simulink subsystem "AutomaticTransmissionWithTorqueConverterSSC"  (R2025b)
settings: Solver=VariableStepAuto  StartTime=0.0  StopTime=10.0  RelTol=1e-3
undefined symbols (not defined in the file): Diff, Eng, PlntTransDampVect, PlntTransEffVect, PlntTransGearNumVect, PlntTransGearRatioVect, PlntTrqConvrtrImpDamp, PlntTrqConvrtrTurbDamp, Trans
libraries: fl_lib x11, sdl_lib x5, nesl_utility x4, nesl_utility_internal x3, autolibsharedcommon x1
settings Model: ModifiedByFormat=The MathWorks, Inc.  Creator=The MathWorks, Inc.  LastModifiedBy=The MathWorks, Inc.
settings OptimizationCC: ReuseModelBlockBuffer=off
settings DebuggingCC: SubsystemReferenceDiagnosticForUnitTest=warning
settings RTWCC: GPUComputeCapability=3.5

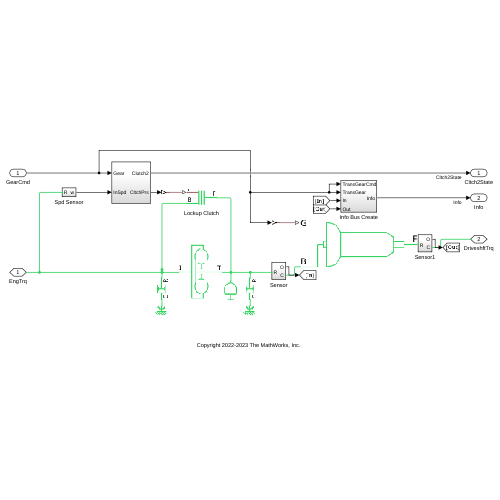
[thumbnail: Simulink's stored preview of the top-level diagram]
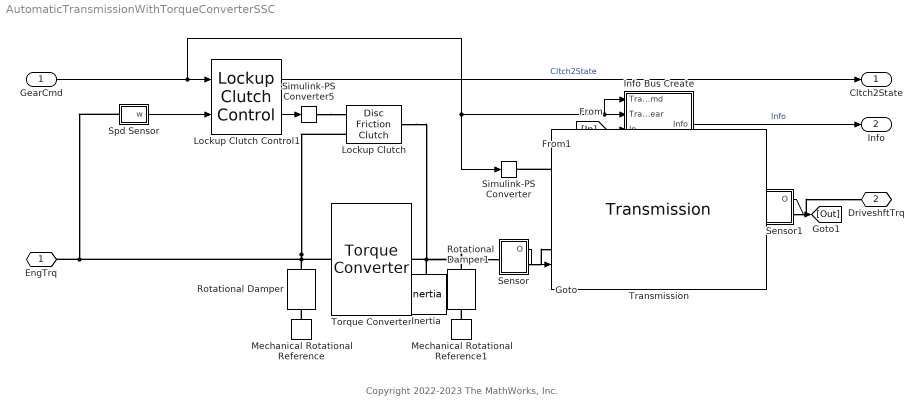
== system AutomaticTransmissionWithTorqueConverterSSC ==
  note: Copyright 2022-2023 The MathWorks, Inc.
  GearCmd : Inport
  Inertia : fl_lib/Mechanical/Rotational Elements/Inertia  inertia=PlntTrqConvrtrTurbInertia kg*m^2  num_ports=foundation.enum.numPorts2.one  w_specify=off  w_priority=High  w=0 rad/s  w_nominal_specify=off  w_nominal_value=1  w_nominal_unit=rad/s  t_specify=off  t_priority=None  t=0 N*m  t_nominal_specify=off  t_nominal_value=1  t_nominal_unit=N*m
  Info Bus Create : Subsystem
  Lockup Clutch : sdl_lib/Clutches/Disc Friction Clutch  geometry_model=sdl.enum.friction_geometry.radius  r_eff=PlntTrqConvrtrCltchRadius m  d_o=150 mm  d_i=100 mm  nS=PlntTrqConvrtrCltchNumFricSurf  piston_area=PlntTrqConvrtrCltchEngdPstnArea m^2  unidirectional=sdl.enum.directionality.bidirectional  friction_model=sdl.enum.friction_model_TLU_thermal.fixed  mu_w_vector=[0, 100, 1000] rad/s  temperature_TLU=[280, 300, 320] K  mu_static=PlntTrqConvrtrCltchStatFric  mu_static_vector=[.4, .38, .36]  mu_coulomb=PlntTrqConvrtrCltchKinFric  mu_coulomb_vector=[.3, .22, .19]  mu_coulomb_temp_vector=[.3, .28, .25]  mu_coulomb_matrix=[.34, .32, .3; .3, .28, .25; .25, .2, .15]  mu_interp_method=simscape.enum.interpolation.linear  mu_extrap_method=simscape.enum.extrapolation.linear  d_f=PlntTrqConvrtrCltchDerateFctr  w_tol=PlntTrqConvrtrCltchVelTol rad/s  pressure_min=PlntTrqConvrtrCltchEngdThreshPrs Pa  mu_visc=PlntTrqConvrtrCltchViscDragTrq N*m/(rad/s)  initial_state_locked=sdl.enum.initial_lock.unlocked  thermal_mass=25 kJ/K  T_init=300 K
      settings: InternalSimscapePortConfiguration="{\"Bottom\":[],\"Left\":[{\"id\":\"P\",\"label\":\"P\",\"type\":\"input\"},{\"id\":\"B\",\"label\":\"B\",\"type\":\"foundation.mechanical.rotational.rotational\"}],\"Right\":[{\"id\":\"F\",\"label\":\"F\",\"type\":\"foundation.mechanical.rotational.rotational\"}],\"Top\":[]}"
  Lockup Clutch Control1 : autolibsharedcommon/Lockup Clutch Control  SystemSampleTime=-1  VariantActivationTime=update diagram  EmptyChoice=off  PassThrough=off  PassThroughVariantControl=(default)  EmptyChoiceVariantControl=(default)  AllowFlexibleInterface=on  Latency=0  AutoFrameSizeCalculation=off
  Mechanical Rotational Reference : fl_lib/Mechanical/Rotational Elements/Mechanical Rotational Reference
  Mechanical Rotational Reference1 : fl_lib/Mechanical/Rotational Elements/Mechanical Rotational Reference
  Rotational Damper : sdl_lib/Couplings & Drives/Springs & Dampers/Rotational Damper  D=PlntTrqConvrtrImpDamp N*m*s/rad  thermal_port=simscape.enum.thermaleffects.omit  thermal_mass=50 kJ/K  temperature_specify=off  temperature_priority=High  temperature=300 K  temperature_nominal_specify=off  temperature_nominal_value=1  temperature_nominal_unit=K
  Rotational Damper1 : sdl_lib/Couplings & Drives/Springs & Dampers/Rotational Damper  D=PlntTrqConvrtrTurbDamp N*m*s/rad  thermal_port=simscape.enum.thermaleffects.omit  thermal_mass=50 kJ/K  temperature_specify=off  temperature_priority=High  temperature=300 K  temperature_nominal_specify=off  temperature_nominal_value=1  temperature_nominal_unit=K
  Sensor : Subsystem
  Sensor1 : Subsystem
  Simulink-PS Converter : nesl_utility_internal/Simulink-PS Converter  PhysicalDomain=network_engine_domain  SubClassName=ps_input  LeftPortType=input  RightPortType=output  PseudoPeriodic=off  Frequencies=[]  NoiseDistribution=none  NoiseParameters=[]  Unit=1  AffineConversion=off  FilteringAndDerivatives=provide  SimscapeFilterOrder=1  InputFilterTimeConstant=0.001  UdotUserProvided=0
  Simulink-PS Converter5 : nesl_utility_internal/Simulink-PS Converter  PhysicalDomain=network_engine_domain  SubClassName=ps_input  LeftPortType=input  RightPortType=output  PseudoPeriodic=off  Frequencies=[]  NoiseDistribution=none  NoiseParameters=[]  Unit=Pa  AffineConversion=off  FilteringAndDerivatives=provide  SimscapeFilterOrder=1  InputFilterTimeConstant=0.01  UdotUserProvided=0
  Spd Sensor : Subsystem
  Torque Converter : sdl_lib/Couplings & Drives/Torque Converter  coast_mode_modeling=sdl.enum.torqueConverterContinuousTwomode.continuous  SR_drive_tlu=PlntTrqConvrtrDrvModeSpdRatioVect  TR_drive_tlu=PlntTrqConvrtrDrvModeTrqRatioVect  CF_drive_tlu=PlntTrqConvrtrDrvModeCapFctrVect N*m/rpm^2  SR_coast_tlu=PlntTrqConvrtrCoastModeSpdRatioVect  CF_coast_tlu=PlntTrqConvrtrCoastModeCapFctrRatioVect N*m/rpm^2  iniMode=sdl.enum.torqueConverterInitialMode.drive  delta_w=PlntTrqConvrtrModeTransThresh rpm  n_vector=PlntTrqConvrtrSpdRatioVect  trq_vector=PlntTrqConvrtrTrqRatioVect  cf_vector_parameterization=sdl.enum.torqueConverterCFParameterization.SpeedToSqrtTorque  cf_vector_reference_speed=sdl.enum.torqueConverterCFReferenceSpeed.ImpellerSpeedAlways  cf_vector=PlntTrqConvrtrCapVect rad/(N^(1/2)*m^(1/2)*s)  cf_vector_sq=1e-3 * [6.616, 6.048, 5.787, 5.384, 4.681, 3.779, 2.671, 2.047, 1.111, .4] N*m*s^2/rad^2  interp_method=simscape.enum.interpolation.smooth  extrap_method=simscape.enum.extrapolation.nearest  model_lag=sdl.enum.torqueConverterLagOnOff.LagOff  tau=PlntTrqConvrtrTimeCnst s  initial_trq_ratio=PlntTrqConvrtrInitTrqRatio
      settings: InternalSimscapePortConfiguration="{\"Bottom\":[],\"Left\":[{\"id\":\"I\",\"label\":\"I\",\"type\":\"foundation.mechanical.rotational.rotational\"}],\"Right\":[{\"id\":\"T\",\"label\":\"T\",\"type\":\"foundation.mechanical.rotational.rotational\"}],\"Top\":[]}"
  Transmission : sdl_lib/Gears/Transmission  gear_ratios=PlntTransGearRatioVect(2:end)  reverse_ratio=PlntTransRvrseGearRatio  friction_model=sdl.enum.transmissionFriction.gear  efficiency=0.95  efficiency_tlu=PlntTransEffVect(2:end)  reverse_efficiency=PlntTransRvrseGearEff  pwr_thr=PlntTransPwrThresh W  kp=PlntTransStiff N*m/rad  kv=PlntTransDamp N*m*s/rad  initial_torque=PlntTransInitInTrq N*m  mu_visc=[PlntTransDampVect(1), PlntTransDampVect(1)] N*m*s/rad  t_friction=PlntTransCltchKinFricTrq N*m  t_locked=PlntTransCltchStatFricTrq N*m  shift_model=sdl.enum.transmissionShiftModel.instant  shift_time=PlntTransCltchShiftTime ms  w_tol=PlntTransCltchVelTol rad/s  initial_state_locked=sdl.enum.initial_lock.locked  thermal_port=simscape.enum.thermaleffects.omit  thermal_mass=100 kJ/K  initial_temperature=300 K
      settings: LogSimulationData=on  InternalSimscapePortConfiguration="{\"Bottom\":[],\"Left\":[{\"id\":\"G\",\"label\":\"G\",\"type\":\"input\"},{\"id\":\"B\",\"label\":\"B\",\"type\":\"foundation.mechanical.rotational.rotational\"}],\"Right\":[{\"id\":\"F\",\"label\":\"F\",\"type\":\"foundation.mechanical.rotational.rotational\"}],\"Top\":[]}"
  EngTrq : PMIOPort  Side=Left
  DriveshftTrq : PMIOPort  Port=2  Side=Right
  Cltch2State : Outport  VectorParamsAs1DForOutWhenUnconnected=off
  Info : Outport  Port=2  VectorParamsAs1DForOutWhenUnconnected=off
  wires:
  Info Bus Create/1(Info) -> Info/1  "Info"
  Lockup Clutch Control1/1 -> Cltch2State/1  "Cltch2State"
  GearCmd/1 -> Lockup Clutch Control1/1, Info Bus Create/2(TransGear), Info Bus Create/1(TransGearCmd), Simulink-PS Converter/1
  Lockup Clutch Control1/2 -> Simulink-PS Converter5/1
  Spd Sensor/1(w) -> Lockup Clutch Control1/2
  Sensor/1(O) -> [In]
  Sensor1/1(O) -> [Out]
  [In] -> Info Bus Create/3(In)
  [Out] -> Info Bus Create/4(Out)
  connections:
  Lockup Clutch/LConn2 -- EngTrq/RConn1 -- Spd Sensor/LConn1 -- Torque Converter/LConn1 -- Rotational Damper/LConn1
  Lockup Clutch/RConn1 -- Sensor/LConn1 -- Rotational Damper1/LConn1 -- Torque Converter/RConn1 -- Inertia/LConn1
  Transmission/LConn1 -- Simulink-PS Converter/RConn1
  Mechanical Rotational Reference/LConn1 -- Rotational Damper/RConn1
  Mechanical Rotational Reference1/LConn1 -- Rotational Damper1/RConn1
  Simulink-PS Converter5/RConn1 -- Lockup Clutch/LConn1
  Sensor1/LConn1 -- Transmission/RConn1
  Sensor/RConn1 -- Transmission/LConn2
  Sensor1/RConn1 -- DriveshftTrq/RConn1

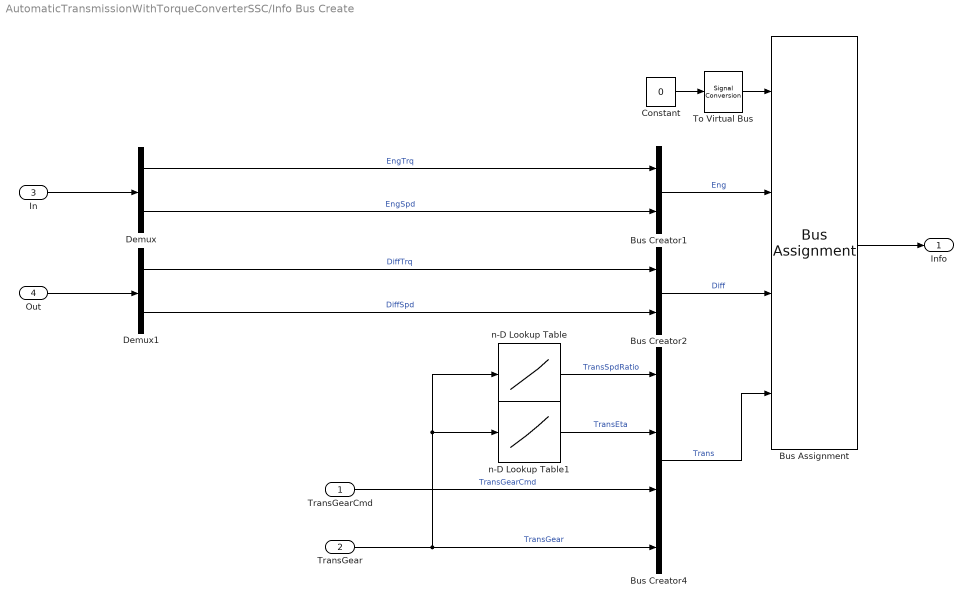
== system AutomaticTransmissionWithTorqueConverterSSC/Info Bus Create ==
  TransGearCmd : Inport
  TransGear : Inport  Port=2
  In : Inport  Port=3
  Out : Inport  Port=4
  Bus Assignment : BusAssignment  AssignedSignals=Eng,Diff,Trans
  Bus Creator1 : BusCreator  Inputs=2
  Bus Creator2 : BusCreator  Inputs=2
  Bus Creator4 : BusCreator  Inputs=4
  Constant : Constant  Value=0  OutDataTypeStr=Bus: InfoBUS  SampleTime=Inf
  Demux : Demux  Outputs=2
  Demux1 : Demux  Outputs=2
  To Virtual Bus : SignalConversion  ConversionOutput=Virtual bus  OverrideOpt=off
  n-D Lookup Table : Lookup_n-D  NumberOfTableDimensions=1  BreakpointsForDimension1=PlntTransGearNumVect  BreakpointsForDimension3=[5, 7]  BeginIndexSearchUsingPreviousIndexResult=on  Table=PlntTransGearRatioVect  InterpMethod=Nearest  ExtrapMethod=Clip  UseLastTableValue=on  InternalRulePriority=Speed  RndMeth=Simplest
  n-D Lookup Table1 : Lookup_n-D  NumberOfTableDimensions=1  BreakpointsForDimension1=PlntTransGearNumVect  BreakpointsForDimension3=[5, 7]  BeginIndexSearchUsingPreviousIndexResult=on  Table=PlntTransEffVect  InterpMethod=Nearest  ExtrapMethod=Clip  UseLastTableValue=on  InternalRulePriority=Speed  RndMeth=Simplest
  Info : Outport
  wires:
  To Virtual Bus/1 -> Bus Assignment/1
  Bus Assignment/1 -> Info/1
  Constant/1 -> To Virtual Bus/1
  Bus Creator2/1 -> Bus Assignment/3  "Diff"
  TransGear/1 -> Bus Creator4/4, n-D Lookup Table1/1, n-D Lookup Table/1  "TransGear"
  Demux/1 -> Bus Creator1/1  "EngTrq"
  n-D Lookup Table/1 -> Bus Creator4/1  "TransSpdRatio"
  Demux1/1 -> Bus Creator2/1  "DiffTrq"
  Demux/2 -> Bus Creator1/2  "EngSpd"
  Bus Creator1/1 -> Bus Assignment/2  "Eng"
  n-D Lookup Table1/1 -> Bus Creator4/2  "TransEta"
  Demux1/2 -> Bus Creator2/2  "DiffSpd"
  Bus Creator4/1 -> Bus Assignment/4  "Trans"
  In/1 -> Demux/1
  Out/1 -> Demux1/1
  TransGearCmd/1 -> Bus Creator4/3  "TransGearCmd"

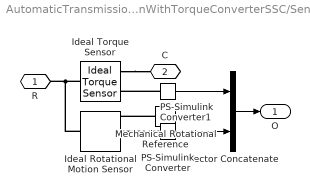
== system AutomaticTransmissionWithTorqueConverterSSC/Sensor ==
  Ideal Rotational Motion Sensor : fl_lib/Mechanical/Mechanical Sensors/Ideal Rotational Motion Sensor  reference=foundation.enum.MeasurementReference.difference  acceleration_port=false  velocity_port=true  position_port=true  wrap_angle=false  offset=0 rad
  Ideal Torque Sensor : fl_lib/Mechanical/Mechanical Sensors/Ideal Torque Sensor
  Mechanical Rotational Reference : fl_lib/Mechanical/Rotational Elements/Mechanical Rotational Reference
  PS-Simulink Converter : nesl_utility/PS-Simulink Converter  PhysicalDomain=network_engine_domain  SubClassName=ps_output  LeftPortType=input  RightPortType=output  PseudoPeriodic=off  Frequencies=[]  VectorFormat=inherit  Unit=inherit  AffineConversion=off
  PS-Simulink Converter1 : nesl_utility/PS-Simulink Converter  PhysicalDomain=network_engine_domain  SubClassName=ps_output  LeftPortType=input  RightPortType=output  PseudoPeriodic=off  Frequencies=[]  VectorFormat=inherit  Unit=inherit  AffineConversion=off
  Vector Concatenate : Concatenate
  R : PMIOPort  Side=Left
  C : PMIOPort  Port=2  Side=Right
  O : Outport
  wires:
  PS-Simulink Converter1/1 -> Vector Concatenate/1
  PS-Simulink Converter/1 -> Vector Concatenate/2
  Vector Concatenate/1 -> O/1
  connections:
  PS-Simulink Converter1/LConn1 -- Ideal Torque Sensor/RConn2
  Ideal Torque Sensor/LConn1 -- Ideal Rotational Motion Sensor/LConn1 -- R/RConn1
  Ideal Torque Sensor/RConn1 -- C/RConn1
  Mechanical Rotational Reference/LConn1 -- Ideal Rotational Motion Sensor/RConn1
  PS-Simulink Converter/LConn1 -- Ideal Rotational Motion Sensor/RConn2

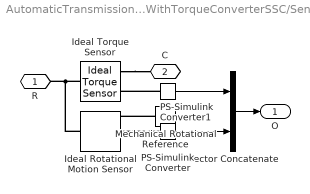
== system AutomaticTransmissionWithTorqueConverterSSC/Sensor1 ==
  Ideal Rotational Motion Sensor : fl_lib/Mechanical/Mechanical Sensors/Ideal Rotational Motion Sensor  reference=foundation.enum.MeasurementReference.difference  acceleration_port=false  velocity_port=true  position_port=true  wrap_angle=false  offset=0 rad
  Ideal Torque Sensor : fl_lib/Mechanical/Mechanical Sensors/Ideal Torque Sensor
  Mechanical Rotational Reference : fl_lib/Mechanical/Rotational Elements/Mechanical Rotational Reference
  PS-Simulink Converter : nesl_utility/PS-Simulink Converter  PhysicalDomain=network_engine_domain  SubClassName=ps_output  LeftPortType=input  RightPortType=output  PseudoPeriodic=off  Frequencies=[]  VectorFormat=inherit  Unit=inherit  AffineConversion=off
  PS-Simulink Converter1 : nesl_utility/PS-Simulink Converter  PhysicalDomain=network_engine_domain  SubClassName=ps_output  LeftPortType=input  RightPortType=output  PseudoPeriodic=off  Frequencies=[]  VectorFormat=inherit  Unit=inherit  AffineConversion=off
  Vector Concatenate : Concatenate
  R : PMIOPort  Side=Left
  C : PMIOPort  Port=2  Side=Right
  O : Outport
  wires:
  Vector Concatenate/1 -> O/1
  PS-Simulink Converter/1 -> Vector Concatenate/2
  PS-Simulink Converter1/1 -> Vector Concatenate/1
  connections:
  PS-Simulink Converter/LConn1 -- Ideal Rotational Motion Sensor/RConn2
  Mechanical Rotational Reference/LConn1 -- Ideal Rotational Motion Sensor/RConn1
  Ideal Torque Sensor/RConn1 -- C/RConn1
  Ideal Rotational Motion Sensor/LConn1 -- Ideal Torque Sensor/LConn1 -- R/RConn1
  PS-Simulink Converter1/LConn1 -- Ideal Torque Sensor/RConn2

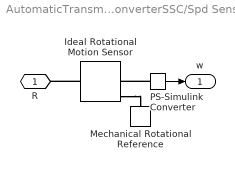
== system AutomaticTransmissionWithTorqueConverterSSC/Spd Sensor ==
  Ideal Rotational Motion Sensor : fl_lib/Mechanical/Mechanical Sensors/Ideal Rotational Motion Sensor  reference=foundation.enum.MeasurementReference.difference  acceleration_port=false  velocity_port=true  position_port=true  wrap_angle=simscape.enum.onoff.off  offset=0 rad
  Mechanical Rotational Reference : fl_lib/Mechanical/Rotational Elements/Mechanical Rotational Reference
  PS-Simulink Converter : nesl_utility_internal/PS-Simulink Converter  PhysicalDomain=network_engine_domain  SubClassName=ps_output  LeftPortType=input  RightPortType=output  PseudoPeriodic=off  Frequencies=[]  VectorFormat=inherit  Unit=inherit  AffineConversion=off
  R : PMIOPort  Side=Left
  w : Outport
  wires:
  PS-Simulink Converter/1 -> w/1
  connections:
  PS-Simulink Converter/LConn1 -- Ideal Rotational Motion Sensor/RConn2
  Ideal Rotational Motion Sensor/LConn1 -- R/RConn1
  Ideal Rotational Motion Sensor/RConn1 -- Mechanical Rotational Reference/LConn1
